simulink model "aes_impl_decrypt_smc"  (R2015b)
settings: Solver=FixedStepDiscrete  SolverMode=SingleTasking  StartTime=0.0  StopTime=1000e-6  RelTol=1e-3
undefined symbols (not defined in the file): a, b, input_sample_rate
libraries: shlslibv1 x3018
(part 2 of 20)

== system aes_impl_decrypt_smc/Round13 ==
  In1 : Inport
  In2 : Inport  Port=2
  In3 : Inport  Port=3
  In4 : Inport  Port=4
  In5 : Inport  Port=5
  In6 : Inport  Port=6
  In7 : Inport  Port=7
  In8 : Inport  Port=8
  In9 : Inport  Port=9
  In10 : Inport  Port=10
  In11 : Inport  Port=11
  In12 : Inport  Port=12
  In13 : Inport  Port=13
  In14 : Inport  Port=14
  In15 : Inport  Port=15
  In16 : Inport  Port=16
  In17 : Inport  Port=17
  In18 : Inport  Port=18
  In19 : Inport  Port=19
  In20 : Inport  Port=20
  In21 : Inport  Port=21
  In22 : Inport  Port=22
  In23 : Inport  Port=23
  In24 : Inport  Port=24
  In25 : Inport  Port=25
  In26 : Inport  Port=26
  In27 : Inport  Port=27
  In28 : Inport  Port=28
  In29 : Inport  Port=29
  In30 : Inport  Port=30
  In31 : Inport  Port=31
  In32 : Inport  Port=32
  Subsystem : Subsystem
  Subsystem8 : Subsystem
  Out1 : Outport
  Out2 : Outport  Port=2
  Out3 : Outport  Port=3
  Out4 : Outport  Port=4
  Out5 : Outport  Port=5
  Out6 : Outport  Port=6
  Out7 : Outport  Port=7
  Out8 : Outport  Port=8
  Out9 : Outport  Port=9
  Out10 : Outport  Port=10
  Out11 : Outport  Port=11
  Out12 : Outport  Port=12
  Out13 : Outport  Port=13
  Out14 : Outport  Port=14
  Out15 : Outport  Port=15
  Out16 : Outport  Port=16
  wires:
  Subsystem/14(Out14) -> Out14/1
  Subsystem/6(Out6) -> Out6/1
  Subsystem/13(Out13) -> Out13/1
  Subsystem/10(Out10) -> Out10/1
  Subsystem/5(Out5) -> Out5/1
  Subsystem/1(Out1) -> Out1/1
  Subsystem/7(Out7) -> Out7/1
  Subsystem/8(Out8) -> Out8/1
  Subsystem/3(Out3) -> Out3/1
  Subsystem/2(Out2) -> Out2/1
  Subsystem/16(Out16) -> Out16/1
  Subsystem/9(Out9) -> Out9/1
  Subsystem/12(Out12) -> Out12/1
  Subsystem/15(Out15) -> Out15/1
  Subsystem/4(Out4) -> Out4/1
  Subsystem/11(Out11) -> Out11/1
  In1/1 -> Subsystem8/1(In1)
  In3/1 -> Subsystem8/3(In3)
  In2/1 -> Subsystem8/2(In2)
  In4/1 -> Subsystem8/4(In4)
  In5/1 -> Subsystem8/5(In5)
  In7/1 -> Subsystem8/7(In7)
  In6/1 -> Subsystem8/6(In6)
  In9/1 -> Subsystem8/9(In9)
  In8/1 -> Subsystem8/8(In8)
  In12/1 -> Subsystem8/12(In12)
  In10/1 -> Subsystem8/10(In10)
  In11/1 -> Subsystem8/11(In11)
  In14/1 -> Subsystem8/14(In14)
  In13/1 -> Subsystem8/13(In13)
  In15/1 -> Subsystem8/15(In15)
  In16/1 -> Subsystem8/16(In16)
  Subsystem8/1(Out1) -> Subsystem/1(In1)
  Subsystem8/2(Out2) -> Subsystem/2(In2)
  Subsystem8/4(Out4) -> Subsystem/4(In4)
  Subsystem8/3(Out3) -> Subsystem/3(In3)
  Subsystem8/6(Out6) -> Subsystem/6(In6)
  Subsystem8/5(Out5) -> Subsystem/5(In5)
  Subsystem8/8(Out8) -> Subsystem/8(In8)
  Subsystem8/7(Out7) -> Subsystem/7(In7)
  Subsystem8/10(Out10) -> Subsystem/10(In10)
  Subsystem8/9(Out9) -> Subsystem/9(In9)
  Subsystem8/11(Out11) -> Subsystem/11(In11)
  Subsystem8/12(Out12) -> Subsystem/12(In12)
  Subsystem8/13(Out13) -> Subsystem/13(In13)
  Subsystem8/15(Out15) -> Subsystem/15(In15)
  Subsystem8/14(Out14) -> Subsystem/14(In14)
  Subsystem8/16(Out16) -> Subsystem/16(In16)
  In31/1 -> Subsystem/31(In31)
  In24/1 -> Subsystem/24(In24)
  In23/1 -> Subsystem/23(In23)
  In22/1 -> Subsystem/22(In22)
  In20/1 -> Subsystem/20(In20)
  In21/1 -> Subsystem/21(In21)
  In25/1 -> Subsystem/25(In25)
  In26/1 -> Subsystem/26(In26)
  In27/1 -> Subsystem/27(In27)
  In28/1 -> Subsystem/28(In28)
  In29/1 -> Subsystem/29(In29)
  In30/1 -> Subsystem/30(In30)
  In32/1 -> Subsystem/32(In32)
  In17/1 -> Subsystem/17(In17)
  In18/1 -> Subsystem/18(In18)
  In19/1 -> Subsystem/19(In19)

== system aes_impl_decrypt_smc/Round14 ==
  In1 : Inport
  In2 : Inport  Port=2
  In3 : Inport  Port=3
  In4 : Inport  Port=4
  In5 : Inport  Port=5
  In6 : Inport  Port=6
  In7 : Inport  Port=7
  In8 : Inport  Port=8
  In9 : Inport  Port=9
  In10 : Inport  Port=10
  In11 : Inport  Port=11
  In12 : Inport  Port=12
  In13 : Inport  Port=13
  In14 : Inport  Port=14
  In15 : Inport  Port=15
  In16 : Inport  Port=16
  In17 : Inport  Port=17
  In18 : Inport  Port=18
  In19 : Inport  Port=19
  In20 : Inport  Port=20
  In21 : Inport  Port=21
  In22 : Inport  Port=22
  In23 : Inport  Port=23
  In24 : Inport  Port=24
  In25 : Inport  Port=25
  In26 : Inport  Port=26
  In27 : Inport  Port=27
  In28 : Inport  Port=28
  In29 : Inport  Port=29
  In30 : Inport  Port=30
  In31 : Inport  Port=31
  In32 : Inport  Port=32
  Subsystem : Subsystem
  Subsystem8 : Subsystem
  Out1 : Outport
  Out2 : Outport  Port=2
  Out3 : Outport  Port=3
  Out4 : Outport  Port=4
  Out5 : Outport  Port=5
  Out6 : Outport  Port=6
  Out7 : Outport  Port=7
  Out8 : Outport  Port=8
  Out9 : Outport  Port=9
  Out10 : Outport  Port=10
  Out11 : Outport  Port=11
  Out12 : Outport  Port=12
  Out13 : Outport  Port=13
  Out14 : Outport  Port=14
  Out15 : Outport  Port=15
  Out16 : Outport  Port=16
  wires:
  Subsystem/14(Out14) -> Out14/1
  Subsystem/6(Out6) -> Out6/1
  Subsystem/13(Out13) -> Out13/1
  Subsystem/10(Out10) -> Out10/1
  Subsystem/5(Out5) -> Out5/1
  Subsystem/1(Out1) -> Out1/1
  Subsystem/7(Out7) -> Out7/1
  Subsystem/8(Out8) -> Out8/1
  Subsystem/3(Out3) -> Out3/1
  Subsystem/2(Out2) -> Out2/1
  Subsystem/16(Out16) -> Out16/1
  Subsystem/9(Out9) -> Out9/1
  Subsystem/12(Out12) -> Out12/1
  Subsystem/15(Out15) -> Out15/1
  Subsystem/4(Out4) -> Out4/1
  Subsystem/11(Out11) -> Out11/1
  In1/1 -> Subsystem8/1(In1)
  In3/1 -> Subsystem8/3(In3)
  In2/1 -> Subsystem8/2(In2)
  In4/1 -> Subsystem8/4(In4)
  In5/1 -> Subsystem8/5(In5)
  In7/1 -> Subsystem8/7(In7)
  In6/1 -> Subsystem8/6(In6)
  In9/1 -> Subsystem8/9(In9)
  In8/1 -> Subsystem8/8(In8)
  In12/1 -> Subsystem8/12(In12)
  In10/1 -> Subsystem8/10(In10)
  In11/1 -> Subsystem8/11(In11)
  In14/1 -> Subsystem8/14(In14)
  In13/1 -> Subsystem8/13(In13)
  In15/1 -> Subsystem8/15(In15)
  In16/1 -> Subsystem8/16(In16)
  Subsystem8/1(Out1) -> Subsystem/1(In1)
  Subsystem8/2(Out2) -> Subsystem/2(In2)
  Subsystem8/4(Out4) -> Subsystem/4(In4)
  Subsystem8/3(Out3) -> Subsystem/3(In3)
  Subsystem8/6(Out6) -> Subsystem/6(In6)
  Subsystem8/5(Out5) -> Subsystem/5(In5)
  Subsystem8/8(Out8) -> Subsystem/8(In8)
  Subsystem8/7(Out7) -> Subsystem/7(In7)
  Subsystem8/10(Out10) -> Subsystem/10(In10)
  Subsystem8/9(Out9) -> Subsystem/9(In9)
  Subsystem8/11(Out11) -> Subsystem/11(In11)
  Subsystem8/12(Out12) -> Subsystem/12(In12)
  Subsystem8/13(Out13) -> Subsystem/13(In13)
  Subsystem8/15(Out15) -> Subsystem/15(In15)
  Subsystem8/14(Out14) -> Subsystem/14(In14)
  Subsystem8/16(Out16) -> Subsystem/16(In16)
  In31/1 -> Subsystem/31(In31)
  In24/1 -> Subsystem/24(In24)
  In23/1 -> Subsystem/23(In23)
  In22/1 -> Subsystem/22(In22)
  In20/1 -> Subsystem/20(In20)
  In21/1 -> Subsystem/21(In21)
  In25/1 -> Subsystem/25(In25)
  In26/1 -> Subsystem/26(In26)
  In27/1 -> Subsystem/27(In27)
  In28/1 -> Subsystem/28(In28)
  In29/1 -> Subsystem/29(In29)
  In30/1 -> Subsystem/30(In30)
  In32/1 -> Subsystem/32(In32)
  In17/1 -> Subsystem/17(In17)
  In18/1 -> Subsystem/18(In18)
  In19/1 -> Subsystem/19(In19)

== system aes_impl_decrypt_smc/Round15 ==
  In1 : Inport
  In2 : Inport  Port=2
  In3 : Inport  Port=3
  In4 : Inport  Port=4
  In5 : Inport  Port=5
  In6 : Inport  Port=6
  In7 : Inport  Port=7
  In8 : Inport  Port=8
  In9 : Inport  Port=9
  In10 : Inport  Port=10
  In11 : Inport  Port=11
  In12 : Inport  Port=12
  In13 : Inport  Port=13
  In14 : Inport  Port=14
  In15 : Inport  Port=15
  In16 : Inport  Port=16
  In17 : Inport  Port=17
  In18 : Inport  Port=18
  In19 : Inport  Port=19
  In20 : Inport  Port=20
  In21 : Inport  Port=21
  In22 : Inport  Port=22
  In23 : Inport  Port=23
  In24 : Inport  Port=24
  In25 : Inport  Port=25
  In26 : Inport  Port=26
  In27 : Inport  Port=27
  In28 : Inport  Port=28
  In29 : Inport  Port=29
  In30 : Inport  Port=30
  In31 : Inport  Port=31
  In32 : Inport  Port=32
  Subsystem : Subsystem
  Subsystem8 : Subsystem
  Out1 : Outport
  Out2 : Outport  Port=2
  Out3 : Outport  Port=3
  Out4 : Outport  Port=4
  Out5 : Outport  Port=5
  Out6 : Outport  Port=6
  Out7 : Outport  Port=7
  Out8 : Outport  Port=8
  Out9 : Outport  Port=9
  Out10 : Outport  Port=10
  Out11 : Outport  Port=11
  Out12 : Outport  Port=12
  Out13 : Outport  Port=13
  Out14 : Outport  Port=14
  Out15 : Outport  Port=15
  Out16 : Outport  Port=16
  wires:
  Subsystem/14(Out14) -> Out14/1
  Subsystem/6(Out6) -> Out6/1
  Subsystem/13(Out13) -> Out13/1
  Subsystem/10(Out10) -> Out10/1
  Subsystem/5(Out5) -> Out5/1
  Subsystem/1(Out1) -> Out1/1
  Subsystem/7(Out7) -> Out7/1
  Subsystem/8(Out8) -> Out8/1
  Subsystem/3(Out3) -> Out3/1
  Subsystem/2(Out2) -> Out2/1
  Subsystem/16(Out16) -> Out16/1
  Subsystem/9(Out9) -> Out9/1
  Subsystem/12(Out12) -> Out12/1
  Subsystem/15(Out15) -> Out15/1
  Subsystem/4(Out4) -> Out4/1
  Subsystem/11(Out11) -> Out11/1
  In1/1 -> Subsystem8/1(In1)
  In3/1 -> Subsystem8/3(In3)
  In2/1 -> Subsystem8/2(In2)
  In4/1 -> Subsystem8/4(In4)
  In5/1 -> Subsystem8/5(In5)
  In7/1 -> Subsystem8/7(In7)
  In6/1 -> Subsystem8/6(In6)
  In9/1 -> Subsystem8/9(In9)
  In8/1 -> Subsystem8/8(In8)
  In12/1 -> Subsystem8/12(In12)
  In10/1 -> Subsystem8/10(In10)
  In11/1 -> Subsystem8/11(In11)
  In14/1 -> Subsystem8/14(In14)
  In13/1 -> Subsystem8/13(In13)
  In15/1 -> Subsystem8/15(In15)
  In16/1 -> Subsystem8/16(In16)
  Subsystem8/1(Out1) -> Subsystem/1(In1)
  Subsystem8/2(Out2) -> Subsystem/2(In2)
  Subsystem8/4(Out4) -> Subsystem/4(In4)
  Subsystem8/3(Out3) -> Subsystem/3(In3)
  Subsystem8/6(Out6) -> Subsystem/6(In6)
  Subsystem8/5(Out5) -> Subsystem/5(In5)
  Subsystem8/8(Out8) -> Subsystem/8(In8)
  Subsystem8/7(Out7) -> Subsystem/7(In7)
  Subsystem8/10(Out10) -> Subsystem/10(In10)
  Subsystem8/9(Out9) -> Subsystem/9(In9)
  Subsystem8/11(Out11) -> Subsystem/11(In11)
  Subsystem8/12(Out12) -> Subsystem/12(In12)
  Subsystem8/13(Out13) -> Subsystem/13(In13)
  Subsystem8/15(Out15) -> Subsystem/15(In15)
  Subsystem8/14(Out14) -> Subsystem/14(In14)
  Subsystem8/16(Out16) -> Subsystem/16(In16)
  In31/1 -> Subsystem/31(In31)
  In24/1 -> Subsystem/24(In24)
  In23/1 -> Subsystem/23(In23)
  In22/1 -> Subsystem/22(In22)
  In20/1 -> Subsystem/20(In20)
  In21/1 -> Subsystem/21(In21)
  In25/1 -> Subsystem/25(In25)
  In26/1 -> Subsystem/26(In26)
  In27/1 -> Subsystem/27(In27)
  In28/1 -> Subsystem/28(In28)
  In29/1 -> Subsystem/29(In29)
  In30/1 -> Subsystem/30(In30)
  In32/1 -> Subsystem/32(In32)
  In17/1 -> Subsystem/17(In17)
  In18/1 -> Subsystem/18(In18)
  In19/1 -> Subsystem/19(In19)

== system aes_impl_decrypt_smc/Round16 ==
  In1 : Inport
  In2 : Inport  Port=2
  In3 : Inport  Port=3
  In4 : Inport  Port=4
  In5 : Inport  Port=5
  In6 : Inport  Port=6
  In7 : Inport  Port=7
  In8 : Inport  Port=8
  In9 : Inport  Port=9
  In10 : Inport  Port=10
  In11 : Inport  Port=11
  In12 : Inport  Port=12
  In13 : Inport  Port=13
  In14 : Inport  Port=14
  In15 : Inport  Port=15
  In16 : Inport  Port=16
  In17 : Inport  Port=17
  In18 : Inport  Port=18
  In19 : Inport  Port=19
  In20 : Inport  Port=20
  In21 : Inport  Port=21
  In22 : Inport  Port=22
  In23 : Inport  Port=23
  In24 : Inport  Port=24
  In25 : Inport  Port=25
  In26 : Inport  Port=26
  In27 : Inport  Port=27
  In28 : Inport  Port=28
  In29 : Inport  Port=29
  In30 : Inport  Port=30
  In31 : Inport  Port=31
  In32 : Inport  Port=32
  Subsystem : Subsystem
  Subsystem8 : Subsystem
  Out1 : Outport
  Out2 : Outport  Port=2
  Out3 : Outport  Port=3
  Out4 : Outport  Port=4
  Out5 : Outport  Port=5
  Out6 : Outport  Port=6
  Out7 : Outport  Port=7
  Out8 : Outport  Port=8
  Out9 : Outport  Port=9
  Out10 : Outport  Port=10
  Out11 : Outport  Port=11
  Out12 : Outport  Port=12
  Out13 : Outport  Port=13
  Out14 : Outport  Port=14
  Out15 : Outport  Port=15
  Out16 : Outport  Port=16
  wires:
  Subsystem/14(Out14) -> Out14/1
  Subsystem/6(Out6) -> Out6/1
  Subsystem/13(Out13) -> Out13/1
  Subsystem/10(Out10) -> Out10/1
  Subsystem/5(Out5) -> Out5/1
  Subsystem/1(Out1) -> Out1/1
  Subsystem/7(Out7) -> Out7/1
  Subsystem/8(Out8) -> Out8/1
  Subsystem/3(Out3) -> Out3/1
  Subsystem/2(Out2) -> Out2/1
  Subsystem/16(Out16) -> Out16/1
  Subsystem/9(Out9) -> Out9/1
  Subsystem/12(Out12) -> Out12/1
  Subsystem/15(Out15) -> Out15/1
  Subsystem/4(Out4) -> Out4/1
  Subsystem/11(Out11) -> Out11/1
  In1/1 -> Subsystem8/1(In1)
  In3/1 -> Subsystem8/3(In3)
  In2/1 -> Subsystem8/2(In2)
  In4/1 -> Subsystem8/4(In4)
  In5/1 -> Subsystem8/5(In5)
  In7/1 -> Subsystem8/7(In7)
  In6/1 -> Subsystem8/6(In6)
  In9/1 -> Subsystem8/9(In9)
  In8/1 -> Subsystem8/8(In8)
  In12/1 -> Subsystem8/12(In12)
  In10/1 -> Subsystem8/10(In10)
  In11/1 -> Subsystem8/11(In11)
  In14/1 -> Subsystem8/14(In14)
  In13/1 -> Subsystem8/13(In13)
  In15/1 -> Subsystem8/15(In15)
  In16/1 -> Subsystem8/16(In16)
  Subsystem8/1(Out1) -> Subsystem/1(In1)
  Subsystem8/2(Out2) -> Subsystem/2(In2)
  Subsystem8/4(Out4) -> Subsystem/4(In4)
  Subsystem8/3(Out3) -> Subsystem/3(In3)
  Subsystem8/6(Out6) -> Subsystem/6(In6)
  Subsystem8/5(Out5) -> Subsystem/5(In5)
  Subsystem8/8(Out8) -> Subsystem/8(In8)
  Subsystem8/7(Out7) -> Subsystem/7(In7)
  Subsystem8/10(Out10) -> Subsystem/10(In10)
  Subsystem8/9(Out9) -> Subsystem/9(In9)
  Subsystem8/11(Out11) -> Subsystem/11(In11)
  Subsystem8/12(Out12) -> Subsystem/12(In12)
  Subsystem8/13(Out13) -> Subsystem/13(In13)
  Subsystem8/15(Out15) -> Subsystem/15(In15)
  Subsystem8/14(Out14) -> Subsystem/14(In14)
  Subsystem8/16(Out16) -> Subsystem/16(In16)
  In31/1 -> Subsystem/31(In31)
  In24/1 -> Subsystem/24(In24)
  In23/1 -> Subsystem/23(In23)
  In22/1 -> Subsystem/22(In22)
  In20/1 -> Subsystem/20(In20)
  In21/1 -> Subsystem/21(In21)
  In25/1 -> Subsystem/25(In25)
  In26/1 -> Subsystem/26(In26)
  In27/1 -> Subsystem/27(In27)
  In28/1 -> Subsystem/28(In28)
  In29/1 -> Subsystem/29(In29)
  In30/1 -> Subsystem/30(In30)
  In32/1 -> Subsystem/32(In32)
  In17/1 -> Subsystem/17(In17)
  In18/1 -> Subsystem/18(In18)
  In19/1 -> Subsystem/19(In19)

== system aes_impl_decrypt_smc/Round17 ==
  In1 : Inport
  In2 : Inport  Port=2
  In3 : Inport  Port=3
  In4 : Inport  Port=4
  In5 : Inport  Port=5
  In6 : Inport  Port=6
  In7 : Inport  Port=7
  In8 : Inport  Port=8
  In9 : Inport  Port=9
  In10 : Inport  Port=10
  In11 : Inport  Port=11
  In12 : Inport  Port=12
  In13 : Inport  Port=13
  In14 : Inport  Port=14
  In15 : Inport  Port=15
  In16 : Inport  Port=16
  In17 : Inport  Port=17
  In18 : Inport  Port=18
  In19 : Inport  Port=19
  In20 : Inport  Port=20
  In21 : Inport  Port=21
  In22 : Inport  Port=22
  In23 : Inport  Port=23
  In24 : Inport  Port=24
  In25 : Inport  Port=25
  In26 : Inport  Port=26
  In27 : Inport  Port=27
  In28 : Inport  Port=28
  In29 : Inport  Port=29
  In30 : Inport  Port=30
  In31 : Inport  Port=31
  In32 : Inport  Port=32
  Subsystem : Subsystem
  Subsystem8 : Subsystem
  Out1 : Outport
  Out2 : Outport  Port=2
  Out3 : Outport  Port=3
  Out4 : Outport  Port=4
  Out5 : Outport  Port=5
  Out6 : Outport  Port=6
  Out7 : Outport  Port=7
  Out8 : Outport  Port=8
  Out9 : Outport  Port=9
  Out10 : Outport  Port=10
  Out11 : Outport  Port=11
  Out12 : Outport  Port=12
  Out13 : Outport  Port=13
  Out14 : Outport  Port=14
  Out15 : Outport  Port=15
  Out16 : Outport  Port=16
  wires:
  Subsystem/14(Out14) -> Out14/1
  Subsystem/6(Out6) -> Out6/1
  Subsystem/13(Out13) -> Out13/1
  Subsystem/10(Out10) -> Out10/1
  Subsystem/5(Out5) -> Out5/1
  Subsystem/1(Out1) -> Out1/1
  Subsystem/7(Out7) -> Out7/1
  Subsystem/8(Out8) -> Out8/1
  Subsystem/3(Out3) -> Out3/1
  Subsystem/2(Out2) -> Out2/1
  Subsystem/16(Out16) -> Out16/1
  Subsystem/9(Out9) -> Out9/1
  Subsystem/12(Out12) -> Out12/1
  Subsystem/15(Out15) -> Out15/1
  Subsystem/4(Out4) -> Out4/1
  Subsystem/11(Out11) -> Out11/1
  In1/1 -> Subsystem8/1(In1)
  In3/1 -> Subsystem8/3(In3)
  In2/1 -> Subsystem8/2(In2)
  In4/1 -> Subsystem8/4(In4)
  In5/1 -> Subsystem8/5(In5)
  In7/1 -> Subsystem8/7(In7)
  In6/1 -> Subsystem8/6(In6)
  In9/1 -> Subsystem8/9(In9)
  In8/1 -> Subsystem8/8(In8)
  In12/1 -> Subsystem8/12(In12)
  In10/1 -> Subsystem8/10(In10)
  In11/1 -> Subsystem8/11(In11)
  In14/1 -> Subsystem8/14(In14)
  In13/1 -> Subsystem8/13(In13)
  In15/1 -> Subsystem8/15(In15)
  In16/1 -> Subsystem8/16(In16)
  Subsystem8/1(Out1) -> Subsystem/1(In1)
  Subsystem8/2(Out2) -> Subsystem/2(In2)
  Subsystem8/4(Out4) -> Subsystem/4(In4)
  Subsystem8/3(Out3) -> Subsystem/3(In3)
  Subsystem8/6(Out6) -> Subsystem/6(In6)
  Subsystem8/5(Out5) -> Subsystem/5(In5)
  Subsystem8/8(Out8) -> Subsystem/8(In8)
  Subsystem8/7(Out7) -> Subsystem/7(In7)
  Subsystem8/10(Out10) -> Subsystem/10(In10)
  Subsystem8/9(Out9) -> Subsystem/9(In9)
  Subsystem8/11(Out11) -> Subsystem/11(In11)
  Subsystem8/12(Out12) -> Subsystem/12(In12)
  Subsystem8/13(Out13) -> Subsystem/13(In13)
  Subsystem8/15(Out15) -> Subsystem/15(In15)
  Subsystem8/14(Out14) -> Subsystem/14(In14)
  Subsystem8/16(Out16) -> Subsystem/16(In16)
  In31/1 -> Subsystem/31(In31)
  In24/1 -> Subsystem/24(In24)
  In23/1 -> Subsystem/23(In23)
  In22/1 -> Subsystem/22(In22)
  In20/1 -> Subsystem/20(In20)
  In21/1 -> Subsystem/21(In21)
  In25/1 -> Subsystem/25(In25)
  In26/1 -> Subsystem/26(In26)
  In27/1 -> Subsystem/27(In27)
  In28/1 -> Subsystem/28(In28)
  In29/1 -> Subsystem/29(In29)
  In30/1 -> Subsystem/30(In30)
  In32/1 -> Subsystem/32(In32)
  In17/1 -> Subsystem/17(In17)
  In18/1 -> Subsystem/18(In18)
  In19/1 -> Subsystem/19(In19)

== system aes_impl_decrypt_smc/Round18 ==
  In1 : Inport
  In2 : Inport  Port=2
  In3 : Inport  Port=3
  In4 : Inport  Port=4
  In5 : Inport  Port=5
  In6 : Inport  Port=6
  In7 : Inport  Port=7
  In8 : Inport  Port=8
  In9 : Inport  Port=9
  In10 : Inport  Port=10
  In11 : Inport  Port=11
  In12 : Inport  Port=12
  In13 : Inport  Port=13
  In14 : Inport  Port=14
  In15 : Inport  Port=15
  In16 : Inport  Port=16
  In17 : Inport  Port=17
  In18 : Inport  Port=18
  In19 : Inport  Port=19
  In20 : Inport  Port=20
  In21 : Inport  Port=21
  In22 : Inport  Port=22
  In23 : Inport  Port=23
  In24 : Inport  Port=24
  In25 : Inport  Port=25
  In26 : Inport  Port=26
  In27 : Inport  Port=27
  In28 : Inport  Port=28
  In29 : Inport  Port=29
  In30 : Inport  Port=30
  In31 : Inport  Port=31
  In32 : Inport  Port=32
  Subsystem : Subsystem
  Subsystem8 : Subsystem
  Out1 : Outport
  Out2 : Outport  Port=2
  Out3 : Outport  Port=3
  Out4 : Outport  Port=4
  Out5 : Outport  Port=5
  Out6 : Outport  Port=6
  Out7 : Outport  Port=7
  Out8 : Outport  Port=8
  Out9 : Outport  Port=9
  Out10 : Outport  Port=10
  Out11 : Outport  Port=11
  Out12 : Outport  Port=12
  Out13 : Outport  Port=13
  Out14 : Outport  Port=14
  Out15 : Outport  Port=15
  Out16 : Outport  Port=16
  wires:
  Subsystem/14(Out14) -> Out14/1
  Subsystem/6(Out6) -> Out6/1
  Subsystem/13(Out13) -> Out13/1
  Subsystem/10(Out10) -> Out10/1
  Subsystem/5(Out5) -> Out5/1
  Subsystem/1(Out1) -> Out1/1
  Subsystem/7(Out7) -> Out7/1
  Subsystem/8(Out8) -> Out8/1
  Subsystem/3(Out3) -> Out3/1
  Subsystem/2(Out2) -> Out2/1
  Subsystem/16(Out16) -> Out16/1
  Subsystem/9(Out9) -> Out9/1
  Subsystem/12(Out12) -> Out12/1
  Subsystem/15(Out15) -> Out15/1
  Subsystem/4(Out4) -> Out4/1
  Subsystem/11(Out11) -> Out11/1
  In1/1 -> Subsystem8/1(In1)
  In3/1 -> Subsystem8/3(In3)
  In2/1 -> Subsystem8/2(In2)
  In4/1 -> Subsystem8/4(In4)
  In5/1 -> Subsystem8/5(In5)
  In7/1 -> Subsystem8/7(In7)
  In6/1 -> Subsystem8/6(In6)
  In9/1 -> Subsystem8/9(In9)
  In8/1 -> Subsystem8/8(In8)
  In12/1 -> Subsystem8/12(In12)
  In10/1 -> Subsystem8/10(In10)
  In11/1 -> Subsystem8/11(In11)
  In14/1 -> Subsystem8/14(In14)
  In13/1 -> Subsystem8/13(In13)
  In15/1 -> Subsystem8/15(In15)
  In16/1 -> Subsystem8/16(In16)
  Subsystem8/1(Out1) -> Subsystem/1(In1)
  Subsystem8/2(Out2) -> Subsystem/2(In2)
  Subsystem8/4(Out4) -> Subsystem/4(In4)
  Subsystem8/3(Out3) -> Subsystem/3(In3)
  Subsystem8/6(Out6) -> Subsystem/6(In6)
  Subsystem8/5(Out5) -> Subsystem/5(In5)
  Subsystem8/8(Out8) -> Subsystem/8(In8)
  Subsystem8/7(Out7) -> Subsystem/7(In7)
  Subsystem8/10(Out10) -> Subsystem/10(In10)
  Subsystem8/9(Out9) -> Subsystem/9(In9)
  Subsystem8/11(Out11) -> Subsystem/11(In11)
  Subsystem8/12(Out12) -> Subsystem/12(In12)
  Subsystem8/13(Out13) -> Subsystem/13(In13)
  Subsystem8/15(Out15) -> Subsystem/15(In15)
  Subsystem8/14(Out14) -> Subsystem/14(In14)
  Subsystem8/16(Out16) -> Subsystem/16(In16)
  In31/1 -> Subsystem/31(In31)
  In24/1 -> Subsystem/24(In24)
  In23/1 -> Subsystem/23(In23)
  In22/1 -> Subsystem/22(In22)
  In20/1 -> Subsystem/20(In20)
  In21/1 -> Subsystem/21(In21)
  In25/1 -> Subsystem/25(In25)
  In26/1 -> Subsystem/26(In26)
  In27/1 -> Subsystem/27(In27)
  In28/1 -> Subsystem/28(In28)
  In29/1 -> Subsystem/29(In29)
  In30/1 -> Subsystem/30(In30)
  In32/1 -> Subsystem/32(In32)
  In17/1 -> Subsystem/17(In17)
  In18/1 -> Subsystem/18(In18)
  In19/1 -> Subsystem/19(In19)

== system aes_impl_decrypt_smc/Round19 ==
  In1 : Inport
  In2 : Inport  Port=2
  In3 : Inport  Port=3
  In4 : Inport  Port=4
  In5 : Inport  Port=5
  In6 : Inport  Port=6
  In7 : Inport  Port=7
  In8 : Inport  Port=8
  In9 : Inport  Port=9
  In10 : Inport  Port=10
  In11 : Inport  Port=11
  In12 : Inport  Port=12
  In13 : Inport  Port=13
  In14 : Inport  Port=14
  In15 : Inport  Port=15
  In16 : Inport  Port=16
  In17 : Inport  Port=17
  In18 : Inport  Port=18
  In19 : Inport  Port=19
  In20 : Inport  Port=20
  In21 : Inport  Port=21
  In22 : Inport  Port=22
  In23 : Inport  Port=23
  In24 : Inport  Port=24
  In25 : Inport  Port=25
  In26 : Inport  Port=26
  In27 : Inport  Port=27
  In28 : Inport  Port=28
  In29 : Inport  Port=29
  In30 : Inport  Port=30
  In31 : Inport  Port=31
  In32 : Inport  Port=32
  Subsystem : Subsystem
  Subsystem8 : Subsystem
  Out1 : Outport
  Out2 : Outport  Port=2
  Out3 : Outport  Port=3
  Out4 : Outport  Port=4
  Out5 : Outport  Port=5
  Out6 : Outport  Port=6
  Out7 : Outport  Port=7
  Out8 : Outport  Port=8
  Out9 : Outport  Port=9
  Out10 : Outport  Port=10
  Out11 : Outport  Port=11
  Out12 : Outport  Port=12
  Out13 : Outport  Port=13
  Out14 : Outport  Port=14
  Out15 : Outport  Port=15
  Out16 : Outport  Port=16
  wires:
  Subsystem/14(Out14) -> Out14/1
  Subsystem/6(Out6) -> Out6/1
  Subsystem/13(Out13) -> Out13/1
  Subsystem/10(Out10) -> Out10/1
  Subsystem/5(Out5) -> Out5/1
  Subsystem/1(Out1) -> Out1/1
  Subsystem/7(Out7) -> Out7/1
  Subsystem/8(Out8) -> Out8/1
  Subsystem/3(Out3) -> Out3/1
  Subsystem/2(Out2) -> Out2/1
  Subsystem/16(Out16) -> Out16/1
  Subsystem/9(Out9) -> Out9/1
  Subsystem/12(Out12) -> Out12/1
  Subsystem/15(Out15) -> Out15/1
  Subsystem/4(Out4) -> Out4/1
  Subsystem/11(Out11) -> Out11/1
  In1/1 -> Subsystem8/1(In1)
  In3/1 -> Subsystem8/3(In3)
  In2/1 -> Subsystem8/2(In2)
  In4/1 -> Subsystem8/4(In4)
  In5/1 -> Subsystem8/5(In5)
  In7/1 -> Subsystem8/7(In7)
  In6/1 -> Subsystem8/6(In6)
  In9/1 -> Subsystem8/9(In9)
  In8/1 -> Subsystem8/8(In8)
  In12/1 -> Subsystem8/12(In12)
  In10/1 -> Subsystem8/10(In10)
  In11/1 -> Subsystem8/11(In11)
  In14/1 -> Subsystem8/14(In14)
  In13/1 -> Subsystem8/13(In13)
  In15/1 -> Subsystem8/15(In15)
  In16/1 -> Subsystem8/16(In16)
  Subsystem8/1(Out1) -> Subsystem/1(In1)
  Subsystem8/2(Out2) -> Subsystem/2(In2)
  Subsystem8/4(Out4) -> Subsystem/4(In4)
  Subsystem8/3(Out3) -> Subsystem/3(In3)
  Subsystem8/6(Out6) -> Subsystem/6(In6)
  Subsystem8/5(Out5) -> Subsystem/5(In5)
  Subsystem8/8(Out8) -> Subsystem/8(In8)
  Subsystem8/7(Out7) -> Subsystem/7(In7)
  Subsystem8/10(Out10) -> Subsystem/10(In10)
  Subsystem8/9(Out9) -> Subsystem/9(In9)
  Subsystem8/11(Out11) -> Subsystem/11(In11)
  Subsystem8/12(Out12) -> Subsystem/12(In12)
  Subsystem8/13(Out13) -> Subsystem/13(In13)
  Subsystem8/15(Out15) -> Subsystem/15(In15)
  Subsystem8/14(Out14) -> Subsystem/14(In14)
  Subsystem8/16(Out16) -> Subsystem/16(In16)
  In31/1 -> Subsystem/31(In31)
  In24/1 -> Subsystem/24(In24)
  In23/1 -> Subsystem/23(In23)
  In22/1 -> Subsystem/22(In22)
  In20/1 -> Subsystem/20(In20)
  In21/1 -> Subsystem/21(In21)
  In25/1 -> Subsystem/25(In25)
  In26/1 -> Subsystem/26(In26)
  In27/1 -> Subsystem/27(In27)
  In28/1 -> Subsystem/28(In28)
  In29/1 -> Subsystem/29(In29)
  In30/1 -> Subsystem/30(In30)
  In32/1 -> Subsystem/32(In32)
  In17/1 -> Subsystem/17(In17)
  In18/1 -> Subsystem/18(In18)
  In19/1 -> Subsystem/19(In19)

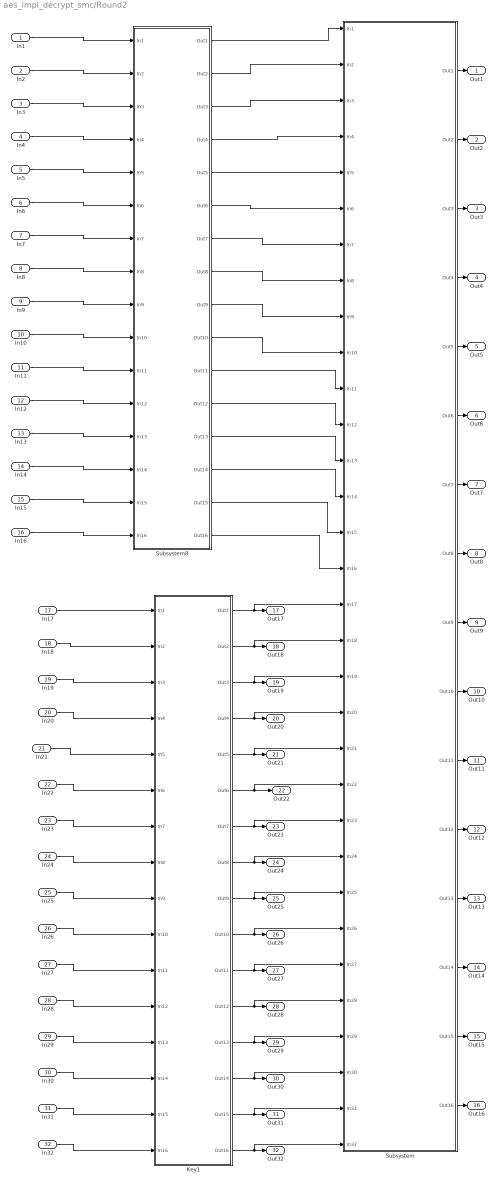
== system aes_impl_decrypt_smc/Round2 ==
  In1 : Inport
  In2 : Inport  Port=2
  In3 : Inport  Port=3
  In4 : Inport  Port=4
  In5 : Inport  Port=5
  In6 : Inport  Port=6
  In7 : Inport  Port=7
  In8 : Inport  Port=8
  In9 : Inport  Port=9
  In10 : Inport  Port=10
  In11 : Inport  Port=11
  In12 : Inport  Port=12
  In13 : Inport  Port=13
  In14 : Inport  Port=14
  In15 : Inport  Port=15
  In16 : Inport  Port=16
  In17 : Inport  Port=17
  In18 : Inport  Port=18
  In19 : Inport  Port=19
  In20 : Inport  Port=20
  In21 : Inport  Port=21
  In22 : Inport  Port=22
  In23 : Inport  Port=23
  In24 : Inport  Port=24
  In25 : Inport  Port=25
  In26 : Inport  Port=26
  In27 : Inport  Port=27
  In28 : Inport  Port=28
  In29 : Inport  Port=29
  In30 : Inport  Port=30
  In31 : Inport  Port=31
  In32 : Inport  Port=32
  Key1 : Subsystem
  Subsystem : Subsystem
  Subsystem8 : Subsystem
  Out1 : Outport
  Out2 : Outport  Port=2
  Out3 : Outport  Port=3
  Out4 : Outport  Port=4
  Out5 : Outport  Port=5
  Out6 : Outport  Port=6
  Out7 : Outport  Port=7
  Out8 : Outport  Port=8
  Out9 : Outport  Port=9
  Out10 : Outport  Port=10
  Out11 : Outport  Port=11
  Out12 : Outport  Port=12
  Out13 : Outport  Port=13
  Out14 : Outport  Port=14
  Out15 : Outport  Port=15
  Out16 : Outport  Port=16
  Out17 : Outport  Port=17
  Out18 : Outport  Port=18
  Out19 : Outport  Port=19
  Out20 : Outport  Port=20
  Out21 : Outport  Port=21
  Out22 : Outport  Port=22
  Out23 : Outport  Port=23
  Out24 : Outport  Port=24
  Out25 : Outport  Port=25
  Out26 : Outport  Port=26
  Out27 : Outport  Port=27
  Out28 : Outport  Port=28
  Out29 : Outport  Port=29
  Out30 : Outport  Port=30
  Out31 : Outport  Port=31
  Out32 : Outport  Port=32
  wires:
  Subsystem/14(Out14) -> Out14/1
  Subsystem/6(Out6) -> Out6/1
  Subsystem/13(Out13) -> Out13/1
  Subsystem/10(Out10) -> Out10/1
  Subsystem/5(Out5) -> Out5/1
  Subsystem/1(Out1) -> Out1/1
  Subsystem/7(Out7) -> Out7/1
  Subsystem/8(Out8) -> Out8/1
  Subsystem/3(Out3) -> Out3/1
  Subsystem/2(Out2) -> Out2/1
  Subsystem/16(Out16) -> Out16/1
  Subsystem/9(Out9) -> Out9/1
  Subsystem/12(Out12) -> Out12/1
  Subsystem/15(Out15) -> Out15/1
  Subsystem/4(Out4) -> Out4/1
  Subsystem/11(Out11) -> Out11/1
  In1/1 -> Subsystem8/1(In1)
  In3/1 -> Subsystem8/3(In3)
  In2/1 -> Subsystem8/2(In2)
  In4/1 -> Subsystem8/4(In4)
  In5/1 -> Subsystem8/5(In5)
  In7/1 -> Subsystem8/7(In7)
  In6/1 -> Subsystem8/6(In6)
  In9/1 -> Subsystem8/9(In9)
  In8/1 -> Subsystem8/8(In8)
  In12/1 -> Subsystem8/12(In12)
  In10/1 -> Subsystem8/10(In10)
  In11/1 -> Subsystem8/11(In11)
  In14/1 -> Subsystem8/14(In14)
  In13/1 -> Subsystem8/13(In13)
  In15/1 -> Subsystem8/15(In15)
  In16/1 -> Subsystem8/16(In16)
  Subsystem8/1(Out1) -> Subsystem/1(In1)
  Subsystem8/2(Out2) -> Subsystem/2(In2)
  Subsystem8/4(Out4) -> Subsystem/4(In4)
  Subsystem8/3(Out3) -> Subsystem/3(In3)
  Subsystem8/6(Out6) -> Subsystem/6(In6)
  Subsystem8/5(Out5) -> Subsystem/5(In5)
  Subsystem8/8(Out8) -> Subsystem/8(In8)
  Subsystem8/7(Out7) -> Subsystem/7(In7)
  Subsystem8/10(Out10) -> Subsystem/10(In10)
  Subsystem8/9(Out9) -> Subsystem/9(In9)
  Subsystem8/11(Out11) -> Subsystem/11(In11)
  Subsystem8/12(Out12) -> Subsystem/12(In12)
  Subsystem8/13(Out13) -> Subsystem/13(In13)
  Subsystem8/15(Out15) -> Subsystem/15(In15)
  Subsystem8/14(Out14) -> Subsystem/14(In14)
  Subsystem8/16(Out16) -> Subsystem/16(In16)
  In17/1 -> Key1/1(In1)
  In19/1 -> Key1/3(In3)
  In18/1 -> Key1/2(In2)
  In21/1 -> Key1/5(In5)
  In20/1 -> Key1/4(In4)
  In23/1 -> Key1/7(In7)
  In22/1 -> Key1/6(In6)
  In25/1 -> Key1/9(In9)
  In24/1 -> Key1/8(In8)
  In27/1 -> Key1/11(In11)
  In26/1 -> Key1/10(In10)
  In29/1 -> Key1/13(In13)
  In28/1 -> Key1/12(In12)
  In30/1 -> Key1/14(In14)
  In31/1 -> Key1/15(In15)
  In32/1 -> Key1/16(In16)
  Key1/14(Out14) -> Out30/1, Subsystem/30(In30)
  Key1/6(Out6) -> Out22/1, Subsystem/22(In22)
  Key1/13(Out13) -> Out29/1, Subsystem/29(In29)
  Key1/10(Out10) -> Out26/1, Subsystem/26(In26)
  Key1/5(Out5) -> Out21/1, Subsystem/21(In21)
  Key1/1(Out1) -> Out17/1, Subsystem/17(In17)
  Key1/7(Out7) -> Out23/1, Subsystem/23(In23)
  Key1/8(Out8) -> Out24/1, Subsystem/24(In24)
  Key1/3(Out3) -> Out19/1, Subsystem/19(In19)
  Key1/2(Out2) -> Out18/1, Subsystem/18(In18)
  Key1/16(Out16) -> Out32/1, Subsystem/32(In32)
  Key1/9(Out9) -> Out25/1, Subsystem/25(In25)
  Key1/12(Out12) -> Out28/1, Subsystem/28(In28)
  Key1/15(Out15) -> Out31/1, Subsystem/31(In31)
  Key1/4(Out4) -> Out20/1, Subsystem/20(In20)
  Key1/11(Out11) -> Out27/1, Subsystem/27(In27)

== system aes_impl_decrypt_smc/Round20 ==
  In1 : Inport
  In2 : Inport  Port=2
  In3 : Inport  Port=3
  In4 : Inport  Port=4
  In5 : Inport  Port=5
  In6 : Inport  Port=6
  In7 : Inport  Port=7
  In8 : Inport  Port=8
  In9 : Inport  Port=9
  In10 : Inport  Port=10
  In11 : Inport  Port=11
  In12 : Inport  Port=12
  In13 : Inport  Port=13
  In14 : Inport  Port=14
  In15 : Inport  Port=15
  In16 : Inport  Port=16
  In17 : Inport  Port=17
  In18 : Inport  Port=18
  In19 : Inport  Port=19
  In20 : Inport  Port=20
  In21 : Inport  Port=21
  In22 : Inport  Port=22
  In23 : Inport  Port=23
  In24 : Inport  Port=24
  In25 : Inport  Port=25
  In26 : Inport  Port=26
  In27 : Inport  Port=27
  In28 : Inport  Port=28
  In29 : Inport  Port=29
  In30 : Inport  Port=30
  In31 : Inport  Port=31
  In32 : Inport  Port=32
  Subsystem : Subsystem
  Subsystem8 : Subsystem
  Out1 : Outport
  Out2 : Outport  Port=2
  Out3 : Outport  Port=3
  Out4 : Outport  Port=4
  Out5 : Outport  Port=5
  Out6 : Outport  Port=6
  Out7 : Outport  Port=7
  Out8 : Outport  Port=8
  Out9 : Outport  Port=9
  Out10 : Outport  Port=10
  Out11 : Outport  Port=11
  Out12 : Outport  Port=12
  Out13 : Outport  Port=13
  Out14 : Outport  Port=14
  Out15 : Outport  Port=15
  Out16 : Outport  Port=16
  wires:
  Subsystem/14(Out14) -> Out14/1
  Subsystem/6(Out6) -> Out6/1
  Subsystem/13(Out13) -> Out13/1
  Subsystem/10(Out10) -> Out10/1
  Subsystem/5(Out5) -> Out5/1
  Subsystem/1(Out1) -> Out1/1
  Subsystem/7(Out7) -> Out7/1
  Subsystem/8(Out8) -> Out8/1
  Subsystem/3(Out3) -> Out3/1
  Subsystem/2(Out2) -> Out2/1
  Subsystem/16(Out16) -> Out16/1
  Subsystem/9(Out9) -> Out9/1
  Subsystem/12(Out12) -> Out12/1
  Subsystem/15(Out15) -> Out15/1
  Subsystem/4(Out4) -> Out4/1
  Subsystem/11(Out11) -> Out11/1
  In1/1 -> Subsystem8/1(In1)
  In3/1 -> Subsystem8/3(In3)
  In2/1 -> Subsystem8/2(In2)
  In4/1 -> Subsystem8/4(In4)
  In5/1 -> Subsystem8/5(In5)
  In7/1 -> Subsystem8/7(In7)
  In6/1 -> Subsystem8/6(In6)
  In9/1 -> Subsystem8/9(In9)
  In8/1 -> Subsystem8/8(In8)
  In12/1 -> Subsystem8/12(In12)
  In10/1 -> Subsystem8/10(In10)
  In11/1 -> Subsystem8/11(In11)
  In14/1 -> Subsystem8/14(In14)
  In13/1 -> Subsystem8/13(In13)
  In15/1 -> Subsystem8/15(In15)
  In16/1 -> Subsystem8/16(In16)
  Subsystem8/1(Out1) -> Subsystem/1(In1)
  Subsystem8/2(Out2) -> Subsystem/2(In2)
  Subsystem8/4(Out4) -> Subsystem/4(In4)
  Subsystem8/3(Out3) -> Subsystem/3(In3)
  Subsystem8/6(Out6) -> Subsystem/6(In6)
  Subsystem8/5(Out5) -> Subsystem/5(In5)
  Subsystem8/8(Out8) -> Subsystem/8(In8)
  Subsystem8/7(Out7) -> Subsystem/7(In7)
  Subsystem8/10(Out10) -> Subsystem/10(In10)
  Subsystem8/9(Out9) -> Subsystem/9(In9)
  Subsystem8/11(Out11) -> Subsystem/11(In11)
  Subsystem8/12(Out12) -> Subsystem/12(In12)
  Subsystem8/13(Out13) -> Subsystem/13(In13)
  Subsystem8/15(Out15) -> Subsystem/15(In15)
  Subsystem8/14(Out14) -> Subsystem/14(In14)
  Subsystem8/16(Out16) -> Subsystem/16(In16)
  In31/1 -> Subsystem/31(In31)
  In24/1 -> Subsystem/24(In24)
  In23/1 -> Subsystem/23(In23)
  In22/1 -> Subsystem/22(In22)
  In20/1 -> Subsystem/20(In20)
  In21/1 -> Subsystem/21(In21)
  In25/1 -> Subsystem/25(In25)
  In26/1 -> Subsystem/26(In26)
  In27/1 -> Subsystem/27(In27)
  In28/1 -> Subsystem/28(In28)
  In29/1 -> Subsystem/29(In29)
  In30/1 -> Subsystem/30(In30)
  In32/1 -> Subsystem/32(In32)
  In17/1 -> Subsystem/17(In17)
  In18/1 -> Subsystem/18(In18)
  In19/1 -> Subsystem/19(In19)

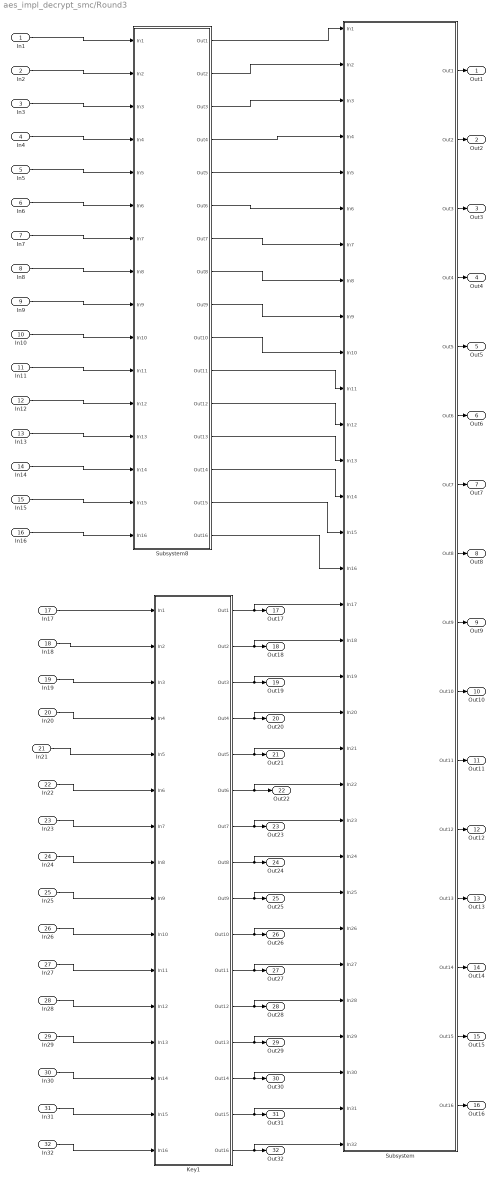
== system aes_impl_decrypt_smc/Round3 ==
  In1 : Inport
  In2 : Inport  Port=2
  In3 : Inport  Port=3
  In4 : Inport  Port=4
  In5 : Inport  Port=5
  In6 : Inport  Port=6
  In7 : Inport  Port=7
  In8 : Inport  Port=8
  In9 : Inport  Port=9
  In10 : Inport  Port=10
  In11 : Inport  Port=11
  In12 : Inport  Port=12
  In13 : Inport  Port=13
  In14 : Inport  Port=14
  In15 : Inport  Port=15
  In16 : Inport  Port=16
  In17 : Inport  Port=17
  In18 : Inport  Port=18
  In19 : Inport  Port=19
  In20 : Inport  Port=20
  In21 : Inport  Port=21
  In22 : Inport  Port=22
  In23 : Inport  Port=23
  In24 : Inport  Port=24
  In25 : Inport  Port=25
  In26 : Inport  Port=26
  In27 : Inport  Port=27
  In28 : Inport  Port=28
  In29 : Inport  Port=29
  In30 : Inport  Port=30
  In31 : Inport  Port=31
  In32 : Inport  Port=32
  Key1 : Subsystem
  Subsystem : Subsystem
  Subsystem8 : Subsystem
  Out1 : Outport
  Out2 : Outport  Port=2
  Out3 : Outport  Port=3
  Out4 : Outport  Port=4
  Out5 : Outport  Port=5
  Out6 : Outport  Port=6
  Out7 : Outport  Port=7
  Out8 : Outport  Port=8
  Out9 : Outport  Port=9
  Out10 : Outport  Port=10
  Out11 : Outport  Port=11
  Out12 : Outport  Port=12
  Out13 : Outport  Port=13
  Out14 : Outport  Port=14
  Out15 : Outport  Port=15
  Out16 : Outport  Port=16
  Out17 : Outport  Port=17
  Out18 : Outport  Port=18
  Out19 : Outport  Port=19
  Out20 : Outport  Port=20
  Out21 : Outport  Port=21
  Out22 : Outport  Port=22
  Out23 : Outport  Port=23
  Out24 : Outport  Port=24
  Out25 : Outport  Port=25
  Out26 : Outport  Port=26
  Out27 : Outport  Port=27
  Out28 : Outport  Port=28
  Out29 : Outport  Port=29
  Out30 : Outport  Port=30
  Out31 : Outport  Port=31
  Out32 : Outport  Port=32
  wires:
  Subsystem/14(Out14) -> Out14/1
  Subsystem/6(Out6) -> Out6/1
  Subsystem/13(Out13) -> Out13/1
  Subsystem/10(Out10) -> Out10/1
  Subsystem/5(Out5) -> Out5/1
  Subsystem/1(Out1) -> Out1/1
  Subsystem/7(Out7) -> Out7/1
  Subsystem/8(Out8) -> Out8/1
  Subsystem/3(Out3) -> Out3/1
  Subsystem/2(Out2) -> Out2/1
  Subsystem/16(Out16) -> Out16/1
  Subsystem/9(Out9) -> Out9/1
  Subsystem/12(Out12) -> Out12/1
  Subsystem/15(Out15) -> Out15/1
  Subsystem/4(Out4) -> Out4/1
  Subsystem/11(Out11) -> Out11/1
  In1/1 -> Subsystem8/1(In1)
  In3/1 -> Subsystem8/3(In3)
  In2/1 -> Subsystem8/2(In2)
  In4/1 -> Subsystem8/4(In4)
  In5/1 -> Subsystem8/5(In5)
  In7/1 -> Subsystem8/7(In7)
  In6/1 -> Subsystem8/6(In6)
  In9/1 -> Subsystem8/9(In9)
  In8/1 -> Subsystem8/8(In8)
  In12/1 -> Subsystem8/12(In12)
  In10/1 -> Subsystem8/10(In10)
  In11/1 -> Subsystem8/11(In11)
  In14/1 -> Subsystem8/14(In14)
  In13/1 -> Subsystem8/13(In13)
  In15/1 -> Subsystem8/15(In15)
  In16/1 -> Subsystem8/16(In16)
  Subsystem8/1(Out1) -> Subsystem/1(In1)
  Subsystem8/2(Out2) -> Subsystem/2(In2)
  Subsystem8/4(Out4) -> Subsystem/4(In4)
  Subsystem8/3(Out3) -> Subsystem/3(In3)
  Subsystem8/6(Out6) -> Subsystem/6(In6)
  Subsystem8/5(Out5) -> Subsystem/5(In5)
  Subsystem8/8(Out8) -> Subsystem/8(In8)
  Subsystem8/7(Out7) -> Subsystem/7(In7)
  Subsystem8/10(Out10) -> Subsystem/10(In10)
  Subsystem8/9(Out9) -> Subsystem/9(In9)
  Subsystem8/11(Out11) -> Subsystem/11(In11)
  Subsystem8/12(Out12) -> Subsystem/12(In12)
  Subsystem8/13(Out13) -> Subsystem/13(In13)
  Subsystem8/15(Out15) -> Subsystem/15(In15)
  Subsystem8/14(Out14) -> Subsystem/14(In14)
  Subsystem8/16(Out16) -> Subsystem/16(In16)
  In17/1 -> Key1/1(In1)
  In19/1 -> Key1/3(In3)
  In18/1 -> Key1/2(In2)
  In21/1 -> Key1/5(In5)
  In20/1 -> Key1/4(In4)
  In23/1 -> Key1/7(In7)
  In22/1 -> Key1/6(In6)
  In25/1 -> Key1/9(In9)
  In24/1 -> Key1/8(In8)
  In27/1 -> Key1/11(In11)
  In26/1 -> Key1/10(In10)
  In29/1 -> Key1/13(In13)
  In28/1 -> Key1/12(In12)
  In30/1 -> Key1/14(In14)
  In31/1 -> Key1/15(In15)
  In32/1 -> Key1/16(In16)
  Key1/14(Out14) -> Out30/1, Subsystem/30(In30)
  Key1/6(Out6) -> Out22/1, Subsystem/22(In22)
  Key1/13(Out13) -> Out29/1, Subsystem/29(In29)
  Key1/10(Out10) -> Out26/1, Subsystem/26(In26)
  Key1/5(Out5) -> Out21/1, Subsystem/21(In21)
  Key1/1(Out1) -> Out17/1, Subsystem/17(In17)
  Key1/7(Out7) -> Out23/1, Subsystem/23(In23)
  Key1/8(Out8) -> Out24/1, Subsystem/24(In24)
  Key1/3(Out3) -> Out19/1, Subsystem/19(In19)
  Key1/2(Out2) -> Out18/1, Subsystem/18(In18)
  Key1/16(Out16) -> Out32/1, Subsystem/32(In32)
  Key1/9(Out9) -> Out25/1, Subsystem/25(In25)
  Key1/12(Out12) -> Out28/1, Subsystem/28(In28)
  Key1/15(Out15) -> Out31/1, Subsystem/31(In31)
  Key1/4(Out4) -> Out20/1, Subsystem/20(In20)
  Key1/11(Out11) -> Out27/1, Subsystem/27(In27)

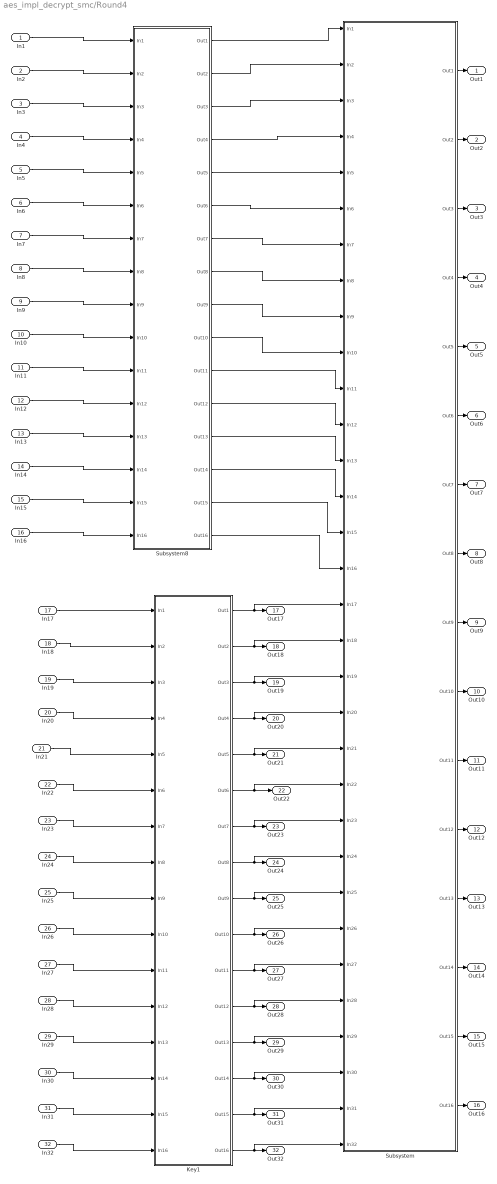
== system aes_impl_decrypt_smc/Round4 ==
  In1 : Inport
  In2 : Inport  Port=2
  In3 : Inport  Port=3
  In4 : Inport  Port=4
  In5 : Inport  Port=5
  In6 : Inport  Port=6
  In7 : Inport  Port=7
  In8 : Inport  Port=8
  In9 : Inport  Port=9
  In10 : Inport  Port=10
  In11 : Inport  Port=11
  In12 : Inport  Port=12
  In13 : Inport  Port=13
  In14 : Inport  Port=14
  In15 : Inport  Port=15
  In16 : Inport  Port=16
  In17 : Inport  Port=17
  In18 : Inport  Port=18
  In19 : Inport  Port=19
  In20 : Inport  Port=20
  In21 : Inport  Port=21
  In22 : Inport  Port=22
  In23 : Inport  Port=23
  In24 : Inport  Port=24
  In25 : Inport  Port=25
  In26 : Inport  Port=26
  In27 : Inport  Port=27
  In28 : Inport  Port=28
  In29 : Inport  Port=29
  In30 : Inport  Port=30
  In31 : Inport  Port=31
  In32 : Inport  Port=32
  Key1 : Subsystem
  Subsystem : Subsystem
  Subsystem8 : Subsystem
  Out1 : Outport
  Out2 : Outport  Port=2
  Out3 : Outport  Port=3
  Out4 : Outport  Port=4
  Out5 : Outport  Port=5
  Out6 : Outport  Port=6
  Out7 : Outport  Port=7
  Out8 : Outport  Port=8
  Out9 : Outport  Port=9
  Out10 : Outport  Port=10
  Out11 : Outport  Port=11
  Out12 : Outport  Port=12
  Out13 : Outport  Port=13
  Out14 : Outport  Port=14
  Out15 : Outport  Port=15
  Out16 : Outport  Port=16
  Out17 : Outport  Port=17
  Out18 : Outport  Port=18
  Out19 : Outport  Port=19
  Out20 : Outport  Port=20
  Out21 : Outport  Port=21
  Out22 : Outport  Port=22
  Out23 : Outport  Port=23
  Out24 : Outport  Port=24
  Out25 : Outport  Port=25
  Out26 : Outport  Port=26
  Out27 : Outport  Port=27
  Out28 : Outport  Port=28
  Out29 : Outport  Port=29
  Out30 : Outport  Port=30
  Out31 : Outport  Port=31
  Out32 : Outport  Port=32
  wires:
  Subsystem/14(Out14) -> Out14/1
  Subsystem/6(Out6) -> Out6/1
  Subsystem/13(Out13) -> Out13/1
  Subsystem/10(Out10) -> Out10/1
  Subsystem/5(Out5) -> Out5/1
  Subsystem/1(Out1) -> Out1/1
  Subsystem/7(Out7) -> Out7/1
  Subsystem/8(Out8) -> Out8/1
  Subsystem/3(Out3) -> Out3/1
  Subsystem/2(Out2) -> Out2/1
  Subsystem/16(Out16) -> Out16/1
  Subsystem/9(Out9) -> Out9/1
  Subsystem/12(Out12) -> Out12/1
  Subsystem/15(Out15) -> Out15/1
  Subsystem/4(Out4) -> Out4/1
  Subsystem/11(Out11) -> Out11/1
  In1/1 -> Subsystem8/1(In1)
  In3/1 -> Subsystem8/3(In3)
  In2/1 -> Subsystem8/2(In2)
  In4/1 -> Subsystem8/4(In4)
  In5/1 -> Subsystem8/5(In5)
  In7/1 -> Subsystem8/7(In7)
  In6/1 -> Subsystem8/6(In6)
  In9/1 -> Subsystem8/9(In9)
  In8/1 -> Subsystem8/8(In8)
  In12/1 -> Subsystem8/12(In12)
  In10/1 -> Subsystem8/10(In10)
  In11/1 -> Subsystem8/11(In11)
  In14/1 -> Subsystem8/14(In14)
  In13/1 -> Subsystem8/13(In13)
  In15/1 -> Subsystem8/15(In15)
  In16/1 -> Subsystem8/16(In16)
  Subsystem8/1(Out1) -> Subsystem/1(In1)
  Subsystem8/2(Out2) -> Subsystem/2(In2)
  Subsystem8/4(Out4) -> Subsystem/4(In4)
  Subsystem8/3(Out3) -> Subsystem/3(In3)
  Subsystem8/6(Out6) -> Subsystem/6(In6)
  Subsystem8/5(Out5) -> Subsystem/5(In5)
  Subsystem8/8(Out8) -> Subsystem/8(In8)
  Subsystem8/7(Out7) -> Subsystem/7(In7)
  Subsystem8/10(Out10) -> Subsystem/10(In10)
  Subsystem8/9(Out9) -> Subsystem/9(In9)
  Subsystem8/11(Out11) -> Subsystem/11(In11)
  Subsystem8/12(Out12) -> Subsystem/12(In12)
  Subsystem8/13(Out13) -> Subsystem/13(In13)
  Subsystem8/15(Out15) -> Subsystem/15(In15)
  Subsystem8/14(Out14) -> Subsystem/14(In14)
  Subsystem8/16(Out16) -> Subsystem/16(In16)
  In17/1 -> Key1/1(In1)
  In19/1 -> Key1/3(In3)
  In18/1 -> Key1/2(In2)
  In21/1 -> Key1/5(In5)
  In20/1 -> Key1/4(In4)
  In23/1 -> Key1/7(In7)
  In22/1 -> Key1/6(In6)
  In25/1 -> Key1/9(In9)
  In24/1 -> Key1/8(In8)
  In27/1 -> Key1/11(In11)
  In26/1 -> Key1/10(In10)
  In29/1 -> Key1/13(In13)
  In28/1 -> Key1/12(In12)
  In30/1 -> Key1/14(In14)
  In31/1 -> Key1/15(In15)
  In32/1 -> Key1/16(In16)
  Key1/14(Out14) -> Out30/1, Subsystem/30(In30)
  Key1/6(Out6) -> Out22/1, Subsystem/22(In22)
  Key1/13(Out13) -> Out29/1, Subsystem/29(In29)
  Key1/10(Out10) -> Out26/1, Subsystem/26(In26)
  Key1/5(Out5) -> Out21/1, Subsystem/21(In21)
  Key1/1(Out1) -> Out17/1, Subsystem/17(In17)
  Key1/7(Out7) -> Out23/1, Subsystem/23(In23)
  Key1/8(Out8) -> Out24/1, Subsystem/24(In24)
  Key1/3(Out3) -> Out19/1, Subsystem/19(In19)
  Key1/2(Out2) -> Out18/1, Subsystem/18(In18)
  Key1/16(Out16) -> Out32/1, Subsystem/32(In32)
  Key1/9(Out9) -> Out25/1, Subsystem/25(In25)
  Key1/12(Out12) -> Out28/1, Subsystem/28(In28)
  Key1/15(Out15) -> Out31/1, Subsystem/31(In31)
  Key1/4(Out4) -> Out20/1, Subsystem/20(In20)
  Key1/11(Out11) -> Out27/1, Subsystem/27(In27)

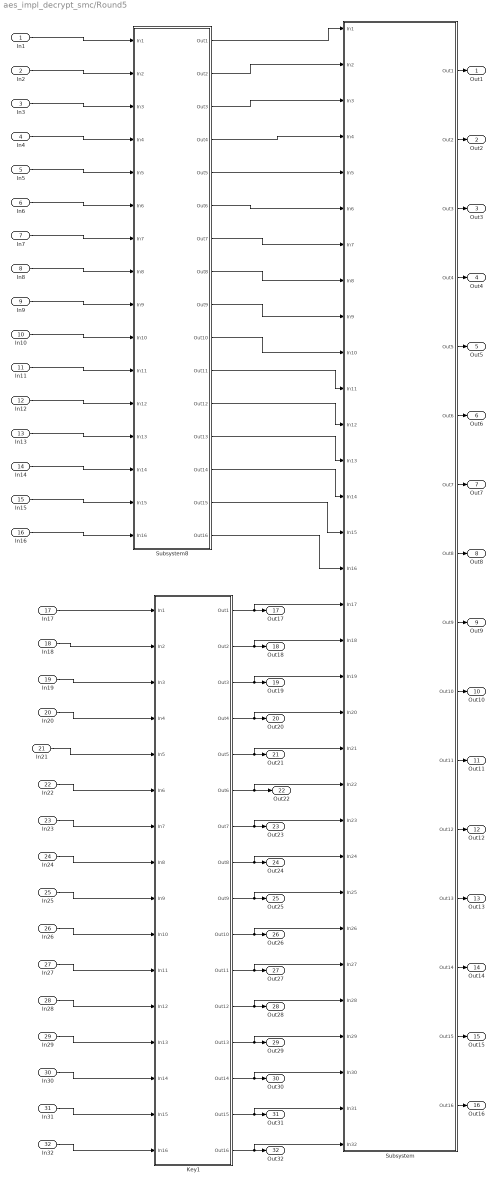
== system aes_impl_decrypt_smc/Round5 ==
  In1 : Inport
  In2 : Inport  Port=2
  In3 : Inport  Port=3
  In4 : Inport  Port=4
  In5 : Inport  Port=5
  In6 : Inport  Port=6
  In7 : Inport  Port=7
  In8 : Inport  Port=8
  In9 : Inport  Port=9
  In10 : Inport  Port=10
  In11 : Inport  Port=11
  In12 : Inport  Port=12
  In13 : Inport  Port=13
  In14 : Inport  Port=14
  In15 : Inport  Port=15
  In16 : Inport  Port=16
  In17 : Inport  Port=17
  In18 : Inport  Port=18
  In19 : Inport  Port=19
  In20 : Inport  Port=20
  In21 : Inport  Port=21
  In22 : Inport  Port=22
  In23 : Inport  Port=23
  In24 : Inport  Port=24
  In25 : Inport  Port=25
  In26 : Inport  Port=26
  In27 : Inport  Port=27
  In28 : Inport  Port=28
  In29 : Inport  Port=29
  In30 : Inport  Port=30
  In31 : Inport  Port=31
  In32 : Inport  Port=32
  Key1 : Subsystem
  Subsystem : Subsystem
  Subsystem8 : Subsystem
  Out1 : Outport
  Out2 : Outport  Port=2
  Out3 : Outport  Port=3
  Out4 : Outport  Port=4
  Out5 : Outport  Port=5
  Out6 : Outport  Port=6
  Out7 : Outport  Port=7
  Out8 : Outport  Port=8
  Out9 : Outport  Port=9
  Out10 : Outport  Port=10
  Out11 : Outport  Port=11
  Out12 : Outport  Port=12
  Out13 : Outport  Port=13
  Out14 : Outport  Port=14
  Out15 : Outport  Port=15
  Out16 : Outport  Port=16
  Out17 : Outport  Port=17
  Out18 : Outport  Port=18
  Out19 : Outport  Port=19
  Out20 : Outport  Port=20
  Out21 : Outport  Port=21
  Out22 : Outport  Port=22
  Out23 : Outport  Port=23
  Out24 : Outport  Port=24
  Out25 : Outport  Port=25
  Out26 : Outport  Port=26
  Out27 : Outport  Port=27
  Out28 : Outport  Port=28
  Out29 : Outport  Port=29
  Out30 : Outport  Port=30
  Out31 : Outport  Port=31
  Out32 : Outport  Port=32
  wires:
  Subsystem/14(Out14) -> Out14/1
  Subsystem/6(Out6) -> Out6/1
  Subsystem/13(Out13) -> Out13/1
  Subsystem/10(Out10) -> Out10/1
  Subsystem/5(Out5) -> Out5/1
  Subsystem/1(Out1) -> Out1/1
  Subsystem/7(Out7) -> Out7/1
  Subsystem/8(Out8) -> Out8/1
  Subsystem/3(Out3) -> Out3/1
  Subsystem/2(Out2) -> Out2/1
  Subsystem/16(Out16) -> Out16/1
  Subsystem/9(Out9) -> Out9/1
  Subsystem/12(Out12) -> Out12/1
  Subsystem/15(Out15) -> Out15/1
  Subsystem/4(Out4) -> Out4/1
  Subsystem/11(Out11) -> Out11/1
  In1/1 -> Subsystem8/1(In1)
  In3/1 -> Subsystem8/3(In3)
  In2/1 -> Subsystem8/2(In2)
  In4/1 -> Subsystem8/4(In4)
  In5/1 -> Subsystem8/5(In5)
  In7/1 -> Subsystem8/7(In7)
  In6/1 -> Subsystem8/6(In6)
  In9/1 -> Subsystem8/9(In9)
  In8/1 -> Subsystem8/8(In8)
  In12/1 -> Subsystem8/12(In12)
  In10/1 -> Subsystem8/10(In10)
  In11/1 -> Subsystem8/11(In11)
  In14/1 -> Subsystem8/14(In14)
  In13/1 -> Subsystem8/13(In13)
  In15/1 -> Subsystem8/15(In15)
  In16/1 -> Subsystem8/16(In16)
  Subsystem8/1(Out1) -> Subsystem/1(In1)
  Subsystem8/2(Out2) -> Subsystem/2(In2)
  Subsystem8/4(Out4) -> Subsystem/4(In4)
  Subsystem8/3(Out3) -> Subsystem/3(In3)
  Subsystem8/6(Out6) -> Subsystem/6(In6)
  Subsystem8/5(Out5) -> Subsystem/5(In5)
  Subsystem8/8(Out8) -> Subsystem/8(In8)
  Subsystem8/7(Out7) -> Subsystem/7(In7)
  Subsystem8/10(Out10) -> Subsystem/10(In10)
  Subsystem8/9(Out9) -> Subsystem/9(In9)
  Subsystem8/11(Out11) -> Subsystem/11(In11)
  Subsystem8/12(Out12) -> Subsystem/12(In12)
  Subsystem8/13(Out13) -> Subsystem/13(In13)
  Subsystem8/15(Out15) -> Subsystem/15(In15)
  Subsystem8/14(Out14) -> Subsystem/14(In14)
  Subsystem8/16(Out16) -> Subsystem/16(In16)
  In17/1 -> Key1/1(In1)
  In19/1 -> Key1/3(In3)
  In18/1 -> Key1/2(In2)
  In21/1 -> Key1/5(In5)
  In20/1 -> Key1/4(In4)
  In23/1 -> Key1/7(In7)
  In22/1 -> Key1/6(In6)
  In25/1 -> Key1/9(In9)
  In24/1 -> Key1/8(In8)
  In27/1 -> Key1/11(In11)
  In26/1 -> Key1/10(In10)
  In29/1 -> Key1/13(In13)
  In28/1 -> Key1/12(In12)
  In30/1 -> Key1/14(In14)
  In31/1 -> Key1/15(In15)
  In32/1 -> Key1/16(In16)
  Key1/14(Out14) -> Out30/1, Subsystem/30(In30)
  Key1/6(Out6) -> Out22/1, Subsystem/22(In22)
  Key1/13(Out13) -> Out29/1, Subsystem/29(In29)
  Key1/10(Out10) -> Out26/1, Subsystem/26(In26)
  Key1/5(Out5) -> Out21/1, Subsystem/21(In21)
  Key1/1(Out1) -> Out17/1, Subsystem/17(In17)
  Key1/7(Out7) -> Out23/1, Subsystem/23(In23)
  Key1/8(Out8) -> Out24/1, Subsystem/24(In24)
  Key1/3(Out3) -> Out19/1, Subsystem/19(In19)
  Key1/2(Out2) -> Out18/1, Subsystem/18(In18)
  Key1/16(Out16) -> Out32/1, Subsystem/32(In32)
  Key1/9(Out9) -> Out25/1, Subsystem/25(In25)
  Key1/12(Out12) -> Out28/1, Subsystem/28(In28)
  Key1/15(Out15) -> Out31/1, Subsystem/31(In31)
  Key1/4(Out4) -> Out20/1, Subsystem/20(In20)
  Key1/11(Out11) -> Out27/1, Subsystem/27(In27)
